simulink model "wcdma_muxandcoding"  (Simulink 6.0)
settings: Solver=FixedStepDiscrete  SolverMode=SingleTasking  StartTime=0.0  StopTime=10.0  RelTol=1e-3
PreLoadFcn:
  | wcdma_loadinitmuxandcoding;
undefined symbols (not defined in the file or in its folder): slcm, totalBitsDelay, trBlkSetSize, tti
libraries: wcdma_lib x16, commrandsrc2 x2, commsink2 x2, dspstat3 x2, commutil2 x1
CloseFcn:
  | % Clear initialization parameters
  | clear RMAttribute numBitsFirstInt numCodeWords posTrCh trBlkSize crcSize numBitsRF  numPadBits slotFormat tti errorCorr numBitsRM numPhCH totalBitsDelay numBitsCodeWord  numBitsTrCh numTrBlks trBlkSetSize
  | 
  | % Clear logging signal
  | clear wcdmaSigsOut
settings Model: Creator=arodrigu  LastModifiedBy=arodrigu  ExtModeAutoUpdateStatusClock=off  ProdHWDeviceType=Specified
settings DataIOCC: LimitDataPoints=off  SaveOutput=off  SaveTime=off  SignalLoggingName=wcdmaSigsOut
settings OptimizationCC: BooleanDataType=off
settings DebuggingCC: CheckExecutionContextPreStartOutputMsg=on  CheckExecutionContextRuntimeOutputMsg=on  SolverPrmCheckMsg=none
settings HardwareCC: ProdHWDeviceType=Specified
settings ModelReferenceCC: UpdateModelReferenceTargets=IfOutOfDate
settings SFSimCC: SFSimApplyToAllLibs=on  SFSimBuildMode=Incremental

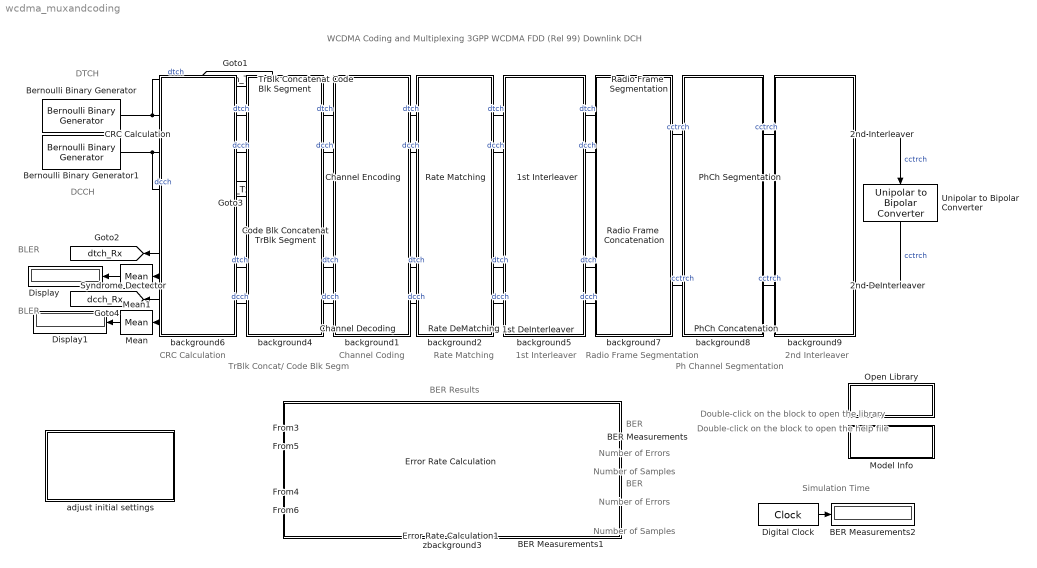
== system wcdma_muxandcoding ==
  note: WCDMA Coding and Multiplexing
      | 3GPP WCDMA FDD (Rel 99) Downlink DCH
  note: Channel
      | Coding
  note: Rate
      | Matching
  note: 1st
      | Interleaver
  note: Radio Frame
      | Segmentation
  note: Ph Channel
      | Segmentation
  note: 2nd
      | Interleaver
  note: DTCH
  note: DCCH
  note: BER
  note: Number of Errors
  note: Number of Samples
  note: BER
  note: Number of Errors
  note: Number of Samples
  note: BER Results
  note: CRC
      | Calculation
  note: TrBlk Concat/
      | Code Blk Segm
  note: BLER
  note: BLER
  note: Simulation Time
  note: Double-click on the block
      | to open the help file
  note: Double-click on the block
      | to open the library
  1st DeInterleaver : wcdma_lib/Wcdma Multiplexing and Channel Coding/1st DeInterleaver  Orientation=left
  1st Interleaver : wcdma_lib/Wcdma Multiplexing and Channel Coding/1st Interleaver
  2nd DeInterleaver : wcdma_lib/Wcdma Multiplexing and Channel Coding/2nd DeInterleaver  Orientation=left
  2nd Interleaver : wcdma_lib/Wcdma Multiplexing and Channel Coding/2nd Interleaver
  BER Measurements : Display
  BER Measurements1 : Display
  BER Measurements2 : Display
  Bernoulli Binary Generator : commrandsrc2/Bernoulli Binary Generator  P=0.5  seed=[123456]  Ts=(tti(1)*1e-3)/trBlkSetSize(1)  frameBased=on  sampPerFrame=trBlkSetSize(1)  orient=off
  Bernoulli Binary Generator1 : commrandsrc2/Bernoulli Binary Generator  P=0.5  seed=[654321]  Ts=(tti(2)*1e-3)/trBlkSetSize(2)  frameBased=on  sampPerFrame=trBlkSetSize(2)  orient=off
  CRC Calculation : wcdma_lib/Wcdma Multiplexing and Channel Coding/CRC Calculation
  Channel Decoding : wcdma_lib/Wcdma Multiplexing and Channel Coding/Channel Decoding  Orientation=left
  Channel Encoding : wcdma_lib/Wcdma Multiplexing and Channel Coding/Channel Encoding
  Code Blk Concatenat TrBlk Segment : wcdma_lib/Wcdma Multiplexing and Channel Coding/Code Blk Concatenat TrBlk Segment  Orientation=left  trBlkSetSize=trBlkSetSize  trBlkSize=trBlkSize  crcSize=crcSize
  Digital Clock : DigitalClock  SampleTime=0.01
  Display : Display
  Display1 : Display
  Error Rate Calculation : commsink2/Error Rate Calculation  N=totalBitsDelay(1)  st_delay=0  cp_mode=Entire frame  subframe=[]  PMode=Port  WsName=ErrorVec  RsMode2=off  stop=off  numErr=100  maxBits=1e6
  Error Rate Calculation1 : commsink2/Error Rate Calculation  N=totalBitsDelay(2)  st_delay=0  cp_mode=Entire frame  subframe=[]  PMode=Port  WsName=ErrorVec  RsMode2=off  stop=off  numErr=100  maxBits=1e6
  Mean : dspstat3/Mean  Orientation=left  DialogController=dspDDGCreate  DialogControllerArgs=DataTag0  run=on  reset_popup=None  roundingMode=Floor  overflowMode=off
  Mean1 : dspstat3/Mean  Orientation=left  DialogController=dspDDGCreate  DialogControllerArgs=DataTag1  run=on  reset_popup=None  roundingMode=Floor  overflowMode=off
  Model Info : Subsystem  LoadFcn=slcm LoadBlock;  InitFcn=slcm('UpdateAllCMBlocksInThisModelInit')  PropExecContextAcrossSSBoundary=on  mask(CMBlock){InitialSaveTempField=, InitialBlockCM=none, BlockCM=none, Frame=on, SaveTempField=, DisplayStringWithTags=Info, MaskDisplayString=Info, HorizontalTextAlignment=Center, LeftAlignmentValue=0.5, SourceBlockDiagram=wcdma_muxandcoding, TagMaxNumber=20, CMTag1=, CMTag2=, CMTag3=, CMTag4=, CMTag5=, CMTag6=, CMTag7=, CMTag8=, CMTag9=, CMTag10=, CMTag11=, CMTag12=, CMTag13=, CMTag14=, CMTag15=, CMTag16=, CMTag17=, CMTag18=, CMTag19=, CMTag20=}
      mask help: This block allows revision control information to be displayed within the model.
      settings: CopyFcn=slcm CopyBlock;  DeleteFcn=slcm Cancel;  PostSaveFcn=slcm('UpdateAllCMBlocksInThisModel')  NameChangeFcn=slcm Rename;  OpenFcn=commdemohelp;
      mask Display: text(str2num(LeftAlignmentValue), 0.5, MaskDisplayString, 'HorizontalAlignment', HorizontalTextAlignment)
  Open Library : Subsystem  PropExecContextAcrossSSBoundary=on
      settings: OpenFcn=open('wcdma_lib.mdl');
      mask Display: disp('WCDMA\nLibrary')
  PhCh Concatenation : wcdma_lib/Wcdma Multiplexing and Channel Coding/PhCh Concatenation  Orientation=left
  PhCh Segmentation : wcdma_lib/Wcdma Multiplexing and Channel Coding/PhCh Segmentation
  Radio Frame  Concatenation : wcdma_lib/Wcdma Multiplexing and Channel Coding/Radio Frame  Concatenation  Orientation=left  numBits=numBitsFirstInt  tti=tti  checkDelay=off
  Radio Frame  Segmentation : wcdma_lib/Wcdma Multiplexing and Channel Coding/Radio Frame  Segmentation
  Rate DeMatching : wcdma_lib/Wcdma Multiplexing and Channel Coding/Rate DeMatching  Orientation=left
  Rate Matching : wcdma_lib/Wcdma Multiplexing and Channel Coding/Rate Matching
  Syndrome Dectector : wcdma_lib/Wcdma Multiplexing and Channel Coding/Syndrome Dectector  Orientation=left
  TrBlk Concatenat Code Blk Segment : wcdma_lib/Wcdma Multiplexing and Channel Coding/TrBlk Concatenat Code Blk Segment  numBitsTrCh=numBitsTrCh  numPadBits=numPadBits  numBitsCodeWord=numBitsCodeWord
  Unipolar to Bipolar Converter : commutil2/Unipolar to Bipolar Converter  Orientation=down  M=2  polarity=Negative
  adjust initial settings : Subsystem  PropExecContextAcrossSSBoundary=on  mask(Wcdma Initial Settings Demo){trBlkSetSize=[732 300], trBlkSize=[244 100], tti=[20 40], crcSize=[16 12], errorCorr=[2 2], RMAttribute=[256 256], posTrCh=0, numPhCH=1, slotFormat=15}
      mask prompts: trBlkSetSize "Transport Block Set Size:"; trBlkSize "Transport Block Size:"; tti "TTI (in ms):"; crcSize "CRC Size {24, 16, 12, 8, 0}:"; errorCorr "Type of Error Protection {None=0, Conv 1/2=1, Conv 1/3=2, Turbo=3}:"; RMAttribute "Rate Matching Attribute:"; posTrCh "Position of TrCH in Radio Frame {Fixed=0, Flexible=1}:"; numPhCH "Number of PhCH:"; slotFormat "Slot Format (0..16):"
      mask help: All the parameters on the mask must be specified as a vector where the k-th element corresponds to the settings for the k-th Transport Channel.
      mask init:
      | numTrBlks = trBlkSetSize./trBlkSize;
      | 
      | % Assign Variables to Workspace
      | assignin('base','trBlkSize',trBlkSize);
      | assignin('base','trBlkSetSize',trBlkSetSize);
      | assignin('base','numTrBlks',numTrBlks);
      | assignin('base','tti',tti);
      | assignin('base','crcSize',crcSize);
      | assignin('base','errorCorr',errorCorr);
      | assignin('base','RMAttribute',RMAttribute);
      | assignin('base','posTrCh',posTrCh);
      | assignin('base','numPhCH',numPhCH);
      | assignin('base','slotFormat',slotFormat);
      | 
      | % Check Params
      | wcdma_checkparamsmuxandcoding;
      | 
      | % Compute Input and Output Ports
      | [numBitsTrCh, numPadBits, numCodeWords, numBitsCodeWord] = wcdma_concseg(trBlkSetSize,trBlkSize,crcSize, errorCorr);
      | assignin('base','numBitsTrCh',numBitsTrCh);
      | assignin('base','numPadBits',numPadBits);
      | assignin('base','numBitsCodeWord',numBitsCodeWord);
      | assignin('base','numCodeWords',numCodeWords);
      | 
      | % Compute Number of Bits at the input of the Rate Matching Block
      | codeRate = errorCorr+1 - (errorCorr == 3);
      | tailBits = 8 *(errorCorr ~=0);
      | numBitsRM = codeRate.*(numBitsCodeWord+tailBits).*numCodeWords;
      | assignin('base','numBitsRM',numBitsRM);
      | 
      | % Compute Number of Bits at the input of the First Interleaver
      | deltaNimax = wcdma_ratematchinginit(numBitsRM, tti, RMAttribute, posTrCh, slotFormat, numPhCH);
      | numBitsFirstInt = numBitsRM + deltaNimax;
      | assignin('base','numBitsFirstInt',numBitsFirstInt);
      | 
      | % Compute number of Bits per Radio Frame
      | numBitsRF = numBitsFirstInt./(tti/10);
      | assignin('base','numBitsRF',numBitsRF);
      | 
      | % Compute Total Delay Tx-Rx
      | totalBitsDelay = (trBlkSetSize.*(1+2*(numCodeWords>1))).*(tti~=10) + (tti==10 & numCodeWords>1)*2.*trBlkSetSize;
      | assignin('base','totalBitsDelay',totalBitsDelay);
      mask Display: disp('Wcdma Demo:\nInitial Settings');
  background1 : Subsystem  PropExecContextAcrossSSBoundary=on
      mask Display: disp('')
  background2 : Subsystem  PropExecContextAcrossSSBoundary=on
      mask Display: disp('')
  background4 : Subsystem  PropExecContextAcrossSSBoundary=on
      mask Display: disp('')
  background5 : Subsystem  PropExecContextAcrossSSBoundary=on
      mask Display: disp('')
  background6 : Subsystem  PropExecContextAcrossSSBoundary=on
      mask Display: disp('')
  background7 : Subsystem  PropExecContextAcrossSSBoundary=on
      mask Display: disp('')
  background8 : Subsystem  PropExecContextAcrossSSBoundary=on
      mask Display: disp('')
  background9 : Subsystem  PropExecContextAcrossSSBoundary=on
      mask Display: disp('')
  zbackground3 : Subsystem  PropExecContextAcrossSSBoundary=on
      mask Display: disp('')
  tag scope: dcch_Rx=global, dcch_Tx=global, dtch_Rx=global, dtch_Tx=global
  wires:
  Bernoulli Binary Generator/1 -> CRC Calculation/1, [dtch_Tx]  "dtch"
  Bernoulli Binary Generator1/1 -> CRC Calculation/2, [dcch_Tx]  "dcch"
  CRC Calculation/1 -> TrBlk Concatenat Code Blk Segment/1  "dtch"
  CRC Calculation/2 -> TrBlk Concatenat Code Blk Segment/2  "dcch"
  TrBlk Concatenat Code Blk Segment/1 -> Channel Encoding/1  "dtch"
  TrBlk Concatenat Code Blk Segment/2 -> Channel Encoding/2  "dcch"
  Rate DeMatching/2 -> Channel Decoding/2  "dcch"
  Channel Encoding/1 -> Rate Matching/1  "dtch"
  Channel Encoding/2 -> Rate Matching/2  "dcch"
  Rate Matching/1 -> 1st Interleaver/1  "dtch"
  Rate Matching/2 -> 1st Interleaver/2  "dcch"
  1st Interleaver/1 -> Radio Frame  Segmentation/1  "dtch"
  1st Interleaver/2 -> Radio Frame  Segmentation/2  "dcch"
  Radio Frame  Segmentation/1 -> PhCh Segmentation/1  "cctrch"
  PhCh Concatenation/1 -> Radio Frame  Concatenation/1  "cctrch"
  PhCh Segmentation/1 -> 2nd Interleaver/1  "cctrch"
  2nd DeInterleaver/1 -> PhCh Concatenation/1  "cctrch"
  Unipolar to Bipolar Converter/1 -> 2nd DeInterleaver/1  "cctrch"
  2nd Interleaver/1 -> Unipolar to Bipolar Converter/1  "cctrch"
  Radio Frame  Concatenation/1 -> 1st DeInterleaver/1  "dtch"
  Radio Frame  Concatenation/2 -> 1st DeInterleaver/2  "dcch"
  1st DeInterleaver/2 -> Rate DeMatching/2  "dcch"
  [dtch_Tx] -> Error Rate Calculation/1
  [dtch_Rx] -> Error Rate Calculation/2
  Error Rate Calculation/1 -> BER Measurements/1
  [dcch_Tx] -> Error Rate Calculation1/1
  [dcch_Rx] -> Error Rate Calculation1/2
  Error Rate Calculation1/1 -> BER Measurements1/1
  Syndrome Dectector/1 -> [dtch_Rx]
  Syndrome Dectector/3 -> [dcch_Rx]
  Syndrome Dectector/2 -> Mean1/1
  Syndrome Dectector/4 -> Mean/1
  Code Blk Concatenat TrBlk Segment/1 -> Syndrome Dectector/1  "dtch"
  Code Blk Concatenat TrBlk Segment/2 -> Syndrome Dectector/2  "dcch"
  Channel Decoding/2 -> Code Blk Concatenat TrBlk Segment/2  "dcch"
  Mean/1 -> Display1/1
  Mean1/1 -> Display/1
  Digital Clock/1 -> BER Measurements2/1
  Channel Decoding/1 -> Code Blk Concatenat TrBlk Segment/1  "dtch"
  Rate DeMatching/1 -> Channel Decoding/1  "dtch"
  1st DeInterleaver/1 -> Rate DeMatching/1  "dtch"

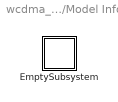
== system wcdma_muxandcoding/Model Info ==
  EmptySubsystem : Subsystem  PropExecContextAcrossSSBoundary=on

== system wcdma_muxandcoding/Open Library ==
  note: This subsystem is intentionally left empty

== system wcdma_muxandcoding/adjust initial settings ==

== system wcdma_muxandcoding/background1 ==

== system wcdma_muxandcoding/background2 ==

== system wcdma_muxandcoding/background4 ==

== system wcdma_muxandcoding/background5 ==

== system wcdma_muxandcoding/background6 ==

== system wcdma_muxandcoding/background7 ==

== system wcdma_muxandcoding/background8 ==

== system wcdma_muxandcoding/background9 ==

== system wcdma_muxandcoding/zbackground3 ==

== system wcdma_muxandcoding/Model Info/EmptySubsystem ==
